simulink model "Kinematik_mit_Getriebe_PT2"  (Simulink 7.1)
settings: Solver=ode5  StartTime=0.0  StopTime=50e-3  FixedStep=1e-6  RelTol=1e-3
undefined symbols (not defined in the file): amplitude, c, d, duty_cycle, duty_on, duty_wert, i, Jc, Jm, komm, komm_start, Mlast, on_time, pwm_on_time, pwm_pause, pwm_periode, pwm_pulse, resolution, wirk
libraries: simulink x1
settings Model: Creator=dep19025415  LastModifiedBy=dep19025415

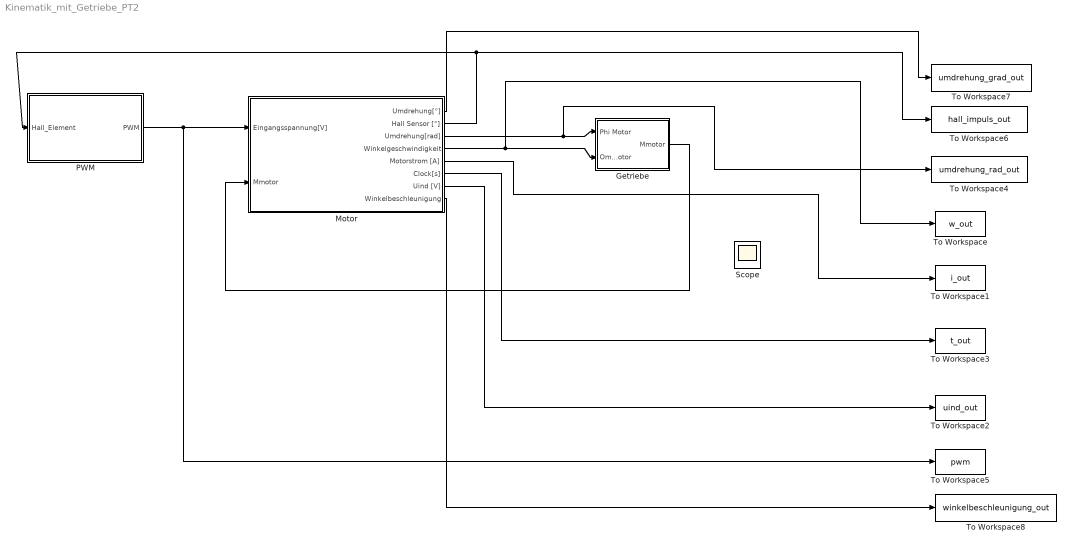
== system Kinematik_mit_Getriebe_PT2 ==
  Getriebe : Subsystem
  Motor : Subsystem
  PWM : Subsystem  mask{ontime=on_time, amp=amplitude, duty=duty_cycle, tpwm=pwm_periode, max=resolution}
      mask prompts: ontime "On time (s)"; amp "Amplitude (V)"; duty "Duty cycle (%)"; tpwm "PWM period (s)"; max "Resolution"
  Scope : Scope  NumInputPorts=2
      settings: YMin=-5~-5  YMax=5~5
  To Workspace : ToWorkspace  VariableName=w_out  SampleTime=-1  SaveFormat=Structure
  To Workspace1 : ToWorkspace  VariableName=i_out  SampleTime=-1  SaveFormat=Structure
  To Workspace2 : ToWorkspace  VariableName=uind_out  SampleTime=-1  SaveFormat=Structure
  To Workspace3 : ToWorkspace  VariableName=t_out  SampleTime=-1  SaveFormat=Structure
  To Workspace4 : ToWorkspace  VariableName=umdrehung_rad_out  SampleTime=-1  SaveFormat=Structure
  To Workspace5 : ToWorkspace  VariableName=pwm  SampleTime=-1  SaveFormat=Structure
  To Workspace6 : ToWorkspace  VariableName=hall_impuls_out  SampleTime=-1  SaveFormat=Structure
  To Workspace7 : ToWorkspace  VariableName=umdrehung_grad_out  SampleTime=-1  SaveFormat=Structure
  To Workspace8 : ToWorkspace  VariableName=winkelbeschleunigung_out  SampleTime=-1  SaveFormat=Structure
  wires:
  PWM/1(PWM) -> Motor/1(Eingangsspannung[V]), To Workspace5/1
  Motor/2(Hall Sensor [°]) -> To Workspace6/1, PWM/1(Hall_Element)
  Motor/3(Umdrehung[rad]) -> Getriebe/1(Phi Motor), To Workspace4/1
  Motor/4(Winkelgeschwindigkeit) -> To Workspace/1, Getriebe/2(Omega Motor)
  Motor/5(Motorstrom [A]) -> To Workspace1/1
  Motor/6(Clock[s]) -> To Workspace3/1
  Motor/7(Uind [V]) -> To Workspace2/1
  Motor/1(Umdrehung[°]) -> To Workspace7/1
  Getriebe/1(Mmotor) -> Motor/2(Mmotor)
  Motor/8(Winkelbeschleunigung) -> To Workspace8/1

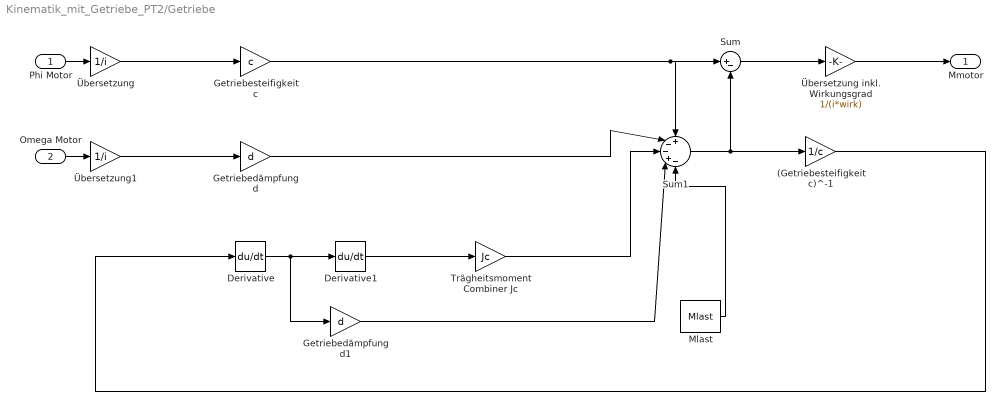
== system Kinematik_mit_Getriebe_PT2/Getriebe ==
  Phi Motor : Inport
  Omega Motor : Inport  Port=2
  (Getriebesteifigkeit c)^-1 : Gain  Gain=1/c  ParameterDataType=sfix(16)  ParameterScaling=2^0  OutDataType=sfix(16)  OutScaling=2^0
  Derivative : Derivative
  Derivative1 : Derivative
  Getriebedämpfung d : Gain  Gain=d  ParameterDataType=sfix(16)  ParameterScaling=2^0  OutDataType=sfix(16)  OutScaling=2^0
  Getriebedämpfung d1 : Gain  Gain=d  ParameterDataType=sfix(16)  ParameterScaling=2^0  OutDataType=sfix(16)  OutScaling=2^0
  Getriebesteifigkeit c : Gain  Gain=c  ParameterDataType=sfix(16)  ParameterScaling=2^0  OutDataType=sfix(16)  OutScaling=2^0
  Mlast : Constant  Value=Mlast  OutDataType=sfix(16)  OutScaling=2^0
  Sum : Sum  Inputs=|+-  OutDataType=sfix(16)  OutScaling=2^0
  Sum1 : Sum  Inputs=+--+-  OutDataType=sfix(16)  OutScaling=2^0
  Trägheitsmoment Combiner Jc : Gain  Gain=Jc  ParameterDataType=sfix(16)  ParameterScaling=2^0  OutDataType=sfix(16)  OutScaling=2^0
  Übersetzung : Gain  Gain=1/i  ParameterDataType=sfix(16)  ParameterScaling=2^0  OutDataType=sfix(16)  OutScaling=2^0
  Übersetzung inkl. Wirkungsgrad : Gain  Gain=1/(i*wirk)  ParameterDataType=sfix(16)  ParameterScaling=2^0  OutDataType=sfix(16)  OutScaling=2^0
  Übersetzung1 : Gain  Gain=1/i  ParameterDataType=sfix(16)  ParameterScaling=2^0  OutDataType=sfix(16)  OutScaling=2^0
  Mmotor : Outport
  wires:
  Übersetzung/1 -> Getriebesteifigkeit c/1
  Übersetzung1/1 -> Getriebedämpfung d/1
  Getriebesteifigkeit c/1 -> Sum/1, Sum1/1
  Getriebedämpfung d/1 -> Sum1/2
  Sum1/1 -> (Getriebesteifigkeit c)^-1/1, Sum/2
  (Getriebesteifigkeit c)^-1/1 -> Derivative/1
  Derivative/1 -> Derivative1/1, Getriebedämpfung d1/1
  Derivative1/1 -> Trägheitsmoment Combiner Jc/1
  Trägheitsmoment Combiner Jc/1 -> Sum1/3
  Getriebedämpfung d1/1 -> Sum1/4
  Mlast/1 -> Sum1/5
  Sum/1 -> Übersetzung inkl. Wirkungsgrad/1
  Phi Motor/1 -> Übersetzung/1
  Übersetzung inkl. Wirkungsgrad/1 -> Mmotor/1
  Omega Motor/1 -> Übersetzung1/1

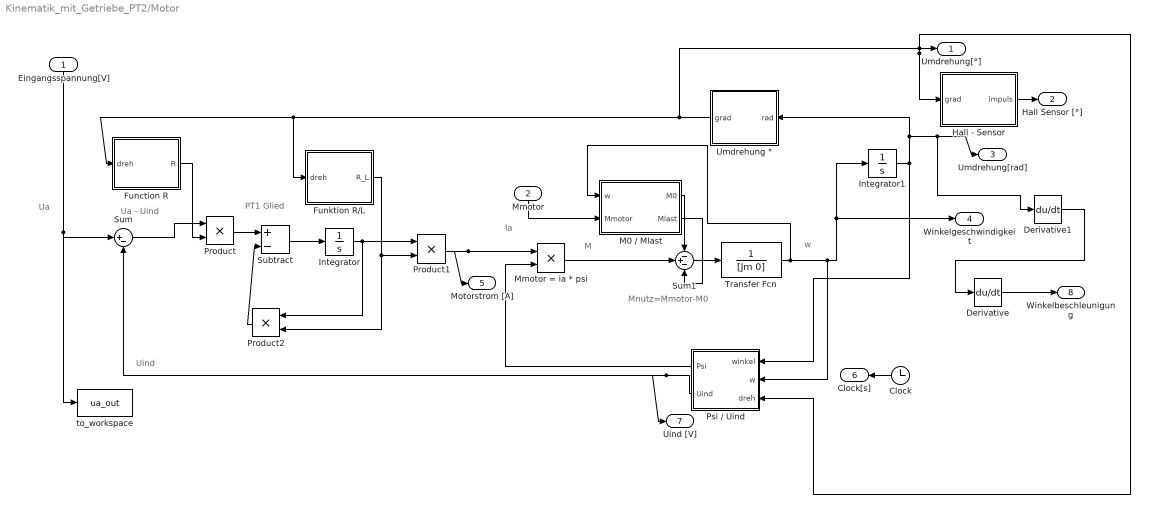
== system Kinematik_mit_Getriebe_PT2/Motor ==
  note: PT1 Glied
  note: M
  note: Ua - Uind
  note: Uind
  note: Ua
  note: Mnutz=Mmotor-M0
  note: Ia
  note: w
  Eingangsspannung[V] : Inport  Orientation=down
  Mmotor : Inport  Orientation=down  Port=2
  Clock : Clock
      settings: Decimation=10
  Derivative : Derivative
  Derivative1 : Derivative
  Function R : Stateflow chart
  Funktion R/L : Stateflow chart
  Hall - Sensor : Stateflow chart
  Integrator : Integrator
  Integrator1 : Integrator
  M0 / Mlast : Stateflow chart
  Mmotor = ia * psi : Product  OutDataType=sfix(16)  OutScaling=2^0  RndMeth=Zero
  Product : Product  OutDataType=sfix(16)  OutScaling=2^0  RndMeth=Zero
  Product1 : Product  OutDataType=sfix(16)  OutScaling=2^0  RndMeth=Zero
  Product2 : Product  Orientation=left  OutDataType=sfix(16)  OutScaling=2^0  RndMeth=Zero
  Psi / Uind : Stateflow chart  Orientation=left
  Subtract : Sum  Inputs=+-  OutDataType=sfix(16)  OutScaling=2^-10
  Sum : Sum  Inputs=|+-  OutDataType=sfix(16)  OutScaling=2^0
  Sum1 : Sum  Inputs=-+-  OutDataType=sfix(16)  OutScaling=2^0
  Transfer Fcn : TransferFcn  Denominator=[Jm 0]
  Umdrehung ° : Stateflow chart  Orientation=left
  to_workspace : ToWorkspace  VariableName=ua_out  SampleTime=-1  SaveFormat=Structure
  Umdrehung[°] : Outport
  Hall Sensor [°] : Outport  Port=2
  Umdrehung[rad] : Outport  Port=3
  Winkelgeschwindigkeit : Outport  Port=4
  Motorstrom [A] : Outport  Port=5
  Clock[s] : Outport  Orientation=left  Port=6
  Uind [V] : Outport  Port=7
  Winkelbeschleunigung : Outport  Port=8
  wires:
  Product1/1 -> Mmotor = ia * psi/1, Motorstrom [A]/1
  Sum/1 -> Product/1
  Umdrehung °/1(grad) -> Funktion R/L/1(dreh), Function R/1(dreh), Umdrehung[°]/1, Hall - Sensor/1(grad), Psi / Uind/3(dreh)
  Psi / Uind/2(Uind) -> Sum/2, Uind [V]/1
  Psi / Uind/1(Psi) -> Mmotor = ia * psi/2
  Mmotor = ia * psi/1 -> Sum1/2
  Integrator1/1 -> Umdrehung °/1(rad), Umdrehung[rad]/1, Derivative1/1, Psi / Uind/1(winkel)
  Transfer Fcn/1 -> Integrator1/1, Winkelgeschwindigkeit/1, Psi / Uind/2(w), M0 / Mlast/1(w)
  Sum1/1 -> Transfer Fcn/1
  Funktion R/L/1(R_L) -> Product1/2, Product2/2
  Function R/1(R) -> Product/2
  Product2/1 -> Subtract/2
  Integrator/1 -> Product1/1, Product2/1
  Subtract/1 -> Integrator/1
  Product/1 -> Subtract/1
  Eingangsspannung[V]/1 -> to_workspace/1, Sum/1
  M0 / Mlast/1(M0) -> Sum1/1
  Hall - Sensor/1(impuls) -> Hall Sensor [°]/1
  Clock/1 -> Clock[s]/1
  M0 / Mlast/2(Mlast) -> Sum1/3
  Mmotor/1 -> M0 / Mlast/2(Mmotor)
  Derivative/1 -> Winkelbeschleunigung/1
  Derivative1/1 -> Derivative/1

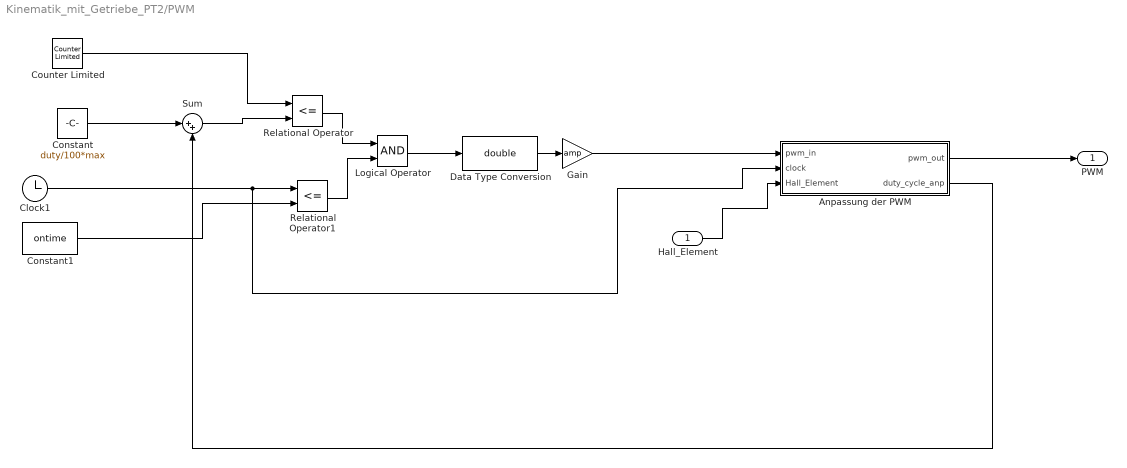
== system Kinematik_mit_Getriebe_PT2/PWM ==
  Hall_Element : Inport  OutDataType=sfix(16)  OutScaling=2^0
  Anpassung der PWM : Stateflow chart
  Clock1 : Clock
      settings: Decimation=10
  Constant : Constant  Value=duty/100*max  OutDataType=sfix(16)  OutScaling=2^0
  Constant1 : Constant  Value=ontime  OutDataType=sfix(16)  OutScaling=2^0
  Counter Limited : simulink/Sources/Counter Limited  SystemSampleTime=-1  uplimit=max  tsamp=tpwm/max
  Data Type Conversion : DataTypeConversion  OutDataTypeMode=double  OutDataType=sfix(16)  OutScaling=2^0  OutDataTypeStr=double
  Gain : Gain  Gain=amp  ParameterDataType=sfix(16)  ParameterScaling=2^0  OutDataType=sfix(16)  OutScaling=2^0
  Logical Operator : Logic  AllPortsSameDT=off  OutDataTypeMode=boolean  OutDataTypeStr=boolean
  Relational Operator : RelationalOperator  Operator=<=  LogicOutDataTypeMode=boolean  OutDataTypeStr=boolean
  Relational Operator1 : RelationalOperator  Operator=<=  LogicOutDataTypeMode=boolean  OutDataTypeStr=boolean
  Sum : Sum  Inputs=|++  OutDataType=sfix(16)  OutScaling=2^0
  PWM : Outport
  wires:
  Counter Limited/1 -> Relational Operator/1
  Clock1/1 -> Relational Operator1/1, Anpassung der PWM/2(clock)
  Constant1/1 -> Relational Operator1/2
  Relational Operator/1 -> Logical Operator/1
  Relational Operator1/1 -> Logical Operator/2
  Logical Operator/1 -> Data Type Conversion/1
  Data Type Conversion/1 -> Gain/1
  Hall_Element/1 -> Anpassung der PWM/3(Hall_Element)
  Gain/1 -> Anpassung der PWM/1(pwm_in)
  Anpassung der PWM/1(pwm_out) -> PWM/1
  Constant/1 -> Sum/1
  Sum/1 -> Relational Operator/2
  Anpassung der PWM/2(duty_cycle_anp) -> Sum/2

== matlab function Motor/M0 / Mlast ==
  data: w input double; M0 output double; Mlast output double; Mmotor input double
function [M0,Mlast] = fcn(w, Mmotor)
% Um zu verhindern, dass die Simulation bei einer Versorgungsspannung von 0V
% den Motor Rückwärts laufen lässt, werden die Reibungsverluste erst ab einem
% sich drehenden Motor berücksichtigt.


M0=0;
Mlast=0;

if w > 0
    M0=0.559e-3;
     Mlast=Mmotor;
end
end

== matlab function Motor/Umdrehung ° ==
  data: rad input double; grad output double
function grad = fcn(rad)
% In dieser Funktion werden die Umdrehung die der Motor sich dreht [in Grad]
% so umgerechnet, dass als Ausgang immer nur Umdrehungen von 0-360° angezeigt
% werden


a = (rad*180/pi)/360;
b = fix(a);
c = a - b;
grad = c * 360;

end

== matlab function Motor/Function R ==
  data: dreh input double; R output double; komm parameter double; komm_start parameter double
function R = fcn(dreh, komm, komm_start)
% In dieser Funktion wird abhängig vom Drehwinkel des Motors der Widerstandswert für R geändert.
% Schließt der Schleifkontakt zwei Kommutierungen kurz, so verringer sich der Widerstand der 
% Drahtwindungen, da eine Spule kurzgeschlossen wird.

R = (1/6.6);
if komm == 1
    if komm_start == 1
        if (dreh >= 60 && dreh <=60.2) || (dreh >= 120 && dreh <= 120.2) || (dreh >= 180 && dreh <= 180.2) || (dreh >= 240 && dreh <= 240.2) || (dreh >= 300 && dreh <= 300.2) || (dreh >= 0 && dreh <= 0.2)
    R = (1/5);
        end
    elseif komm_start == 0
        if (dreh >= 60 && dreh <=60.2) || (dreh >= 120 && dreh <= 120.2) || (dreh >= 180 && dreh <= 180.2) || (dreh >= 240 && dreh <= 240.2) || (dreh >= 300 && dreh <= 300.2)
        R = (1/5);
        end
    end
end
end

== matlab function Motor/Funktion R/L ==
  data: dreh input double; R_L output double; komm parameter double; komm_start parameter double
function R_L = fcn(dreh, komm, komm_start)
% In dieser Funktion wird abhängig vom Drehwinkel des Motors der Wert für R und L geändert.
% Schließt der Schleifkontakt zwei Kommutierungen kurz, so verringer sich der Widerstand, als 
% als auch die Induktivität der Spulen, da eine Spule kurzgeschlossen wird. 


R_L = (6/7.3e-3);
if komm == 1
    if komm_start == 1
        if (dreh >= 60 && dreh <=60.2) || (dreh >= 120 && dreh <= 120.2) || (dreh >= 180 && dreh <= 180.2) || (dreh >= 240 && dreh <= 240.2) || (dreh >= 300 && dreh <= 300.2) || (dreh >= 0 && dreh <= 0.2)
    R_L = (5/5.5e-3);
        end
    elseif komm_start == 0
        if (dreh >= 60 && dreh <=60.2) || (dreh >= 120 && dreh <= 120.2) || (dreh >= 180 && dreh <= 180.2) || (dreh >= 240 && dreh <= 240.2) || (dreh >= 300 && dreh <= 300.2)
        R_L = (5/5.5e-3);
        end
    end
end
end

== matlab function Motor/Psi / Uind ==
  data: winkel input double; w input double; Psi output double; Uind output double; dreh input double; komm parameter double; komm_start parameter double
function [Psi, Uind] = fcn(winkel, w, dreh, komm, komm_start)
% In dieser Funktion wird abhängig von der Drehposition des Motors
% die induzierte Spannung (Uind) als auch der magnetische Verkettete
% Fluss (Psi) berechnet

Uind = nan;
EMF = 5;
psicon = EMF / (100 * pi);

Psi =  psicon * (sin(winkel+pi/3*(1-fix(3/pi*winkel))));

if komm == 1
    if komm_start == 1
        if (dreh >= 60 && dreh <=60.2) || (dreh >= 120 && dreh <= 120.2) || (dreh >= 180 && dreh <= 180.2) || (dreh >= 240 && dreh <= 240.2) || (dreh >= 300 && dreh <= 300.2) || (dreh >= 0 && dreh <= 0.2)
    Psi = Psi * 2 / 3;
        end
    elseif komm_start == 0
        if (dreh >= 60 && dreh <=60.2) || (dreh >= 120 && dreh <= 120.2) || (dreh >= 180 && dreh <= 180.2) || (dreh >= 240 && dreh <= 240.2) || (dreh >= 300 && dreh <= 300.2)
        Psi = Psi * 2 / 3;
        end
    end
end


Uind = (2 * pi / 6) * w * Psi;

end

== matlab function Motor/Hall - Sensor ==
  data: grad input double; impuls output double
function impuls = fcn(grad)
% In dieser Funktion werden die Umdrehung die der Motor sich dreht [in Grad]
% so umgerechnet, dass als Ausgang immer nur Umdrehungen von 0-360° angezeigt
% werden


impuls = nan;
if (grad >=0 && grad <= 22.5)
    impuls = 0;
end
if (grad >=22.5 && grad <= 45)
    impuls = 1;
end
if (grad >=45 && grad <= 67.5)
    impuls = 0;
end
if (grad >=67.5 && grad <= 90)
    impuls = 1;
end
if (grad >=90 && grad <= 112.5)
    impuls = 0;
end
if (grad >=112.5 && grad <= 135)
    impuls = 1;
end
if (grad >=135 && grad <= 157.5)
    impuls = 0;
end
if (grad >=157.5 && grad <= 180)
    impuls = 1;
end
if (grad >=180 && grad <= 202.5)
    impuls = 0;
end
if (grad >=202.5 && grad <= 225)
    impuls = 1;
end
if (grad >=225 && grad <= 247.5)
    impuls = 0;
end
if (grad >=247.5 && grad <= 270)
    impuls = 1;
end
if (grad >=270 && grad <= 292.5)
    impuls = 0;
end
if (grad >=292.5 && grad <= 315)
    impuls = 1;
end
if (grad >=315 && grad <= 337.5)
    impuls = 0;
end
if (grad >=337.5 && grad <= 0)
    impuls = 1;
end


end

== matlab function PWM/Anpassung der PWM ==
  data: pwm_in input double; pwm_out output double; clock input double; Hall_Element input double; pwm_on_time parameter double; pwm_pause parameter double; pwm_pulse parameter double; duty_on parameter double; duty_wert parameter double; amplitude parameter double; duty_cycle_anp output double; max parameter double
function [pwm_out,duty_cycle_anp] = fcn(pwm_in, clock, Hall_Element, pwm_on_time, pwm_pause, pwm_pulse, duty_on, duty_wert, amplitude, max)
% This block supports the Embedded MATLAB subset.
% See the help menu for details. 

pwm_out = pwm_in;
duty_cycle_anp = 0;
a=fix(clock/pwm_on_time);
time = (pwm_pause+pwm_on_time);
b=fix(clock/time);
if duty_on == 0
    duty_cycle_anp = 0;
elseif duty_on == 1
    duty_cycle_anp = ((b)*(duty_wert/100))*max;
end
if pwm_pulse == 1
if Hall_Element == 1
    pwm_out = 0;
else
    if clock >= pwm_on_time && clock <= time
        pwm_out=0;
    end
    if clock >= ((b*time)+pwm_on_time) && clock <= ((b+1)*time)
        pwm_out=0;
    end
end
end

end

    
% if duty_on == 1
%     pwm_out = pwm_in * ((b+1)*duty_wert/100);
%     if pwm_out >= amplitude
%         pwm_out = amplitude;
%     end
